simulink model "frt_e"  (R2012b)
(part 3 of 76)

      |     if (t < 0) || (t > 2),
      |         problem = t;
      |         ctr = numios + 1;
      |     end
      | end
      | if problem ~= 0,
      |     error('Type cannot be %i, must be 0, 1 or 2.', problem);
      | end
      mask Callback bin_pts:
      | blk = gcb;
      | mode = get_param(blk, 'mode');
      | current_bins = eval(get_param(blk, 'bin_pts'));
      | if (strcmp(mode, 'one value') || strcmp(mode, 'fields of equal size')) && (length(current_bins) > 1),
      |     error('Only one binary pt may be specified for this mode.');
      | elseif strcmp(mode, 'fields of arbitrary size')
      |     current_names = textscan(strtrim(strrep(strrep(get_param(blk, 'names'), ']', ''), '[', '')), '%s');
      |     current_names = current_names{1};
      |     numios = length(current_names);
      |     if length(current_bins) ~= numios,
      |         error('%d field names specified, but %d binary pts?', numios, length(current_bins));
      |     end
      | end
  txip3 : Subsystem  Tag=xps:sw_reg  AncestorBlock=xps_library/software register  mask(swreg){mode=one value, io_dir=To Processor, io_delay=0, sample_period=1, names=ip, bitwidths=32, arith_types=0, bin_pts=0, sim_port=off, show_format=on}
      mask prompts: io_dir "I/O direction"; io_delay "I/O delay"; sample_period "Sample period"; names "Name:"; bitwidths "Bitwidth:"; arith_types "Type (ufix=0, fix=1, bool=2):"; bin_pts "Binary pt:"; sim_port "Provide sim input/output?"; show_format "Print format string?"
      mask init:
      | swreg_init(gcb)
      settings: AttributesFormatString=1output:uf32.0,
      mask TypeOptions mode: one value | fields of equal size | fields of arbitrary size
      mask Callback mode: swreg_cb(gcb);
      mask TypeOptions io_dir: To Processor | From Processor
      mask Callback io_dir:
      | mask_enables = get_param(gcb, 'MaskEnables');
      | mask_names = get_param(gcb, 'MaskNames');
      | if strcmp(get_param(gcb, 'io_dir'), 'To Processor'),
      |     mask_enables{ismember(mask_names, 'sample_period')} = 'off';
      | else
      |     mask_enables{ismember(mask_names, 'sample_period')} = 'on';
      | end
      | set_param(gcb, 'MaskEnables', mask_enables);
      mask Callback bitwidths:
      | blk = gcb;
      | mode = get_param(blk, 'mode');
      | current_widths = eval(get_param(blk, 'bitwidths'));
      | if (strcmp(mode, 'one value') || strcmp(mode, 'fields of equal size')) && (length(current_widths) > 1),
      |     error('Only one width may be specified for this mode.');
      | elseif strcmp(mode, 'fields of arbitrary size')
      |     current_names = textscan(strtrim(strrep(strrep(get_param(blk, 'names'), ']', ''), '[', '')), '%s');
      |     current_names = current_names{1};
      |     numios = length(current_names);
      |     if length(current_widths) ~= numios,
      |         error('%d field names specified, but %d widths?', numios, length(current_widths));
      |     end
      | end
      | total_width = 0;
      | for ctr = 1 : length(current_widths),
      |     total_width = total_width + current_widths(ctr);
      | end
      | if total_width > 32,
      |     error('Total width must be 32 or less, set to %d.', total_width);
      | end
      mask Callback arith_types:
      | blk = gcb;
      | mode = get_param(blk, 'mode');
      | current_types = eval(get_param(blk, 'arith_types'));
      | numios = length(current_types);
      | if (strcmp(mode, 'one value') || strcmp(mode, 'fields of equal size')) && (length(current_types) > 1),
      |     error('Only one type may be specified for this mode.');
      | elseif strcmp(mode, 'fields of arbitrary size')
      |     current_names = textscan(strtrim(strrep(strrep(get_param(blk, 'names'), ']', ''), '[', '')), '%s');
      |     current_names = current_names{1};
      |     numios = length(current_names);
      |     if length(current_types) ~= numios,
      |         error('%d field names specified, but %d types?', numios, length(current_types));
      |     end
      | end
      | problem = 0;
      | for ctr = 1 : numios,
      |     t = current_types(ctr);
      |     if (t < 0) || (t > 2),
      |         problem = t;
      |         ctr = numios + 1;
      |     end
      | end
      | if problem ~= 0,
      |     error('Type cannot be %i, must be 0, 1 or 2.', problem);
      | end
      mask Callback bin_pts:
      | blk = gcb;
      | mode = get_param(blk, 'mode');
      | current_bins = eval(get_param(blk, 'bin_pts'));
      | if (strcmp(mode, 'one value') || strcmp(mode, 'fields of equal size')) && (length(current_bins) > 1),
      |     error('Only one binary pt may be specified for this mode.');
      | elseif strcmp(mode, 'fields of arbitrary size')
      |     current_names = textscan(strtrim(strrep(strrep(get_param(blk, 'names'), ']', ''), '[', '')), '%s');
      |     current_names = current_names{1};
      |     numios = length(current_names);
      |     if length(current_bins) ~= numios,
      |         error('%d field names specified, but %d binary pts?', numios, length(current_bins));
      |     end
      | end
  txpport01 : Subsystem  Tag=xps:sw_reg  AncestorBlock=xps_library/software register  mask(swreg){mode=fields of equal size, io_dir=To Processor, io_delay=0, sample_period=1, names=[port0 port1], bitwidths=32/2, arith_types=0, bin_pts=0, sim_port=off, show_format=on}
      mask prompts: io_dir "I/O direction"; io_delay "I/O delay"; sample_period "Sample period"; names "Names [msb ... lsb]:"; bitwidths "Bitwidth:"; arith_types "Type (ufix=0, fix=1, bool=2):"; bin_pts "Binary pt:"; sim_port "Provide sim input/output?"; show_format "Print format string?"
      mask init:
      | swreg_init(gcb)
      settings: AttributesFormatString=2 outputs:uf16.0,uf16.0,
      mask TypeOptions mode: one value | fields of equal size | fields of arbitrary size
      mask Callback mode: swreg_cb(gcb);
      mask TypeOptions io_dir: To Processor | From Processor
      mask Callback io_dir:
      | mask_enables = get_param(gcb, 'MaskEnables');
      | mask_names = get_param(gcb, 'MaskNames');
      | if strcmp(get_param(gcb, 'io_dir'), 'To Processor'),
      |     mask_enables{ismember(mask_names, 'sample_period')} = 'off';
      | else
      |     mask_enables{ismember(mask_names, 'sample_period')} = 'on';
      | end
      | set_param(gcb, 'MaskEnables', mask_enables);
      mask Callback bitwidths:
      | blk = gcb;
      | mode = get_param(blk, 'mode');
      | current_widths = eval(get_param(blk, 'bitwidths'));
      | if (strcmp(mode, 'one value') || strcmp(mode, 'fields of equal size')) && (length(current_widths) > 1),
      |     error('Only one width may be specified for this mode.');
      | elseif strcmp(mode, 'fields of arbitrary size')
      |     current_names = textscan(strtrim(strrep(strrep(get_param(blk, 'names'), ']', ''), '[', '')), '%s');
      |     current_names = current_names{1};
      |     numios = length(current_names);
      |     if length(current_widths) ~= numios,
      |         error('%d field names specified, but %d widths?', numios, length(current_widths));
      |     end
      | end
      | total_width = 0;
      | for ctr = 1 : length(current_widths),
      |     total_width = total_width + current_widths(ctr);
      | end
      | if total_width > 32,
      |     error('Total width must be 32 or less, set to %d.', total_width);
      | end
      mask Callback arith_types:
      | blk = gcb;
      | mode = get_param(blk, 'mode');
      | current_types = eval(get_param(blk, 'arith_types'));
      | numios = length(current_types);
      | if (strcmp(mode, 'one value') || strcmp(mode, 'fields of equal size')) && (length(current_types) > 1),
      |     error('Only one type may be specified for this mode.');
      | elseif strcmp(mode, 'fields of arbitrary size')
      |     current_names = textscan(strtrim(strrep(strrep(get_param(blk, 'names'), ']', ''), '[', '')), '%s');
      |     current_names = current_names{1};
      |     numios = length(current_names);
      |     if length(current_types) ~= numios,
      |         error('%d field names specified, but %d types?', numios, length(current_types));
      |     end
      | end
      | problem = 0;
      | for ctr = 1 : numios,
      |     t = current_types(ctr);
      |     if (t < 0) || (t > 2),
      |         problem = t;
      |         ctr = numios + 1;
      |     end
      | end
      | if problem ~= 0,
      |     error('Type cannot be %i, must be 0, 1 or 2.', problem);
      | end
      mask Callback bin_pts:
      | blk = gcb;
      | mode = get_param(blk, 'mode');
      | current_bins = eval(get_param(blk, 'bin_pts'));
      | if (strcmp(mode, 'one value') || strcmp(mode, 'fields of equal size')) && (length(current_bins) > 1),
      |     error('Only one binary pt may be specified for this mode.');
      | elseif strcmp(mode, 'fields of arbitrary size')
      |     current_names = textscan(strtrim(strrep(strrep(get_param(blk, 'names'), ']', ''), '[', '')), '%s');
      |     current_names = current_names{1};
      |     numios = length(current_names);
      |     if length(current_bins) ~= numios,
      |         error('%d field names specified, but %d binary pts?', numios, length(current_bins));
      |     end
      | end
  txpport23 : Subsystem  Tag=xps:sw_reg  AncestorBlock=xps_library/software register  mask(swreg){mode=fields of equal size, io_dir=To Processor, io_delay=0, sample_period=1, names=[port2 port3], bitwidths=32/2, arith_types=0, bin_pts=0, sim_port=off, show_format=on}
      mask prompts: io_dir "I/O direction"; io_delay "I/O delay"; sample_period "Sample period"; names "Names [msb ... lsb]:"; bitwidths "Bitwidth:"; arith_types "Type (ufix=0, fix=1, bool=2):"; bin_pts "Binary pt:"; sim_port "Provide sim input/output?"; show_format "Print format string?"
      mask init:
      | swreg_init(gcb)
      settings: AttributesFormatString=2 outputs:uf16.0,uf16.0,
      mask TypeOptions mode: one value | fields of equal size | fields of arbitrary size
      mask Callback mode: swreg_cb(gcb);
      mask TypeOptions io_dir: To Processor | From Processor
      mask Callback io_dir:
      | mask_enables = get_param(gcb, 'MaskEnables');
      | mask_names = get_param(gcb, 'MaskNames');
      | if strcmp(get_param(gcb, 'io_dir'), 'To Processor'),
      |     mask_enables{ismember(mask_names, 'sample_period')} = 'off';
      | else
      |     mask_enables{ismember(mask_names, 'sample_period')} = 'on';
      | end
      | set_param(gcb, 'MaskEnables', mask_enables);
      mask Callback bitwidths:
      | blk = gcb;
      | mode = get_param(blk, 'mode');
      | current_widths = eval(get_param(blk, 'bitwidths'));
      | if (strcmp(mode, 'one value') || strcmp(mode, 'fields of equal size')) && (length(current_widths) > 1),
      |     error('Only one width may be specified for this mode.');
      | elseif strcmp(mode, 'fields of arbitrary size')
      |     current_names = textscan(strtrim(strrep(strrep(get_param(blk, 'names'), ']', ''), '[', '')), '%s');
      |     current_names = current_names{1};
      |     numios = length(current_names);
      |     if length(current_widths) ~= numios,
      |         error('%d field names specified, but %d widths?', numios, length(current_widths));
      |     end
      | end
      | total_width = 0;
      | for ctr = 1 : length(current_widths),
      |     total_width = total_width + current_widths(ctr);
      | end
      | if total_width > 32,
      |     error('Total width must be 32 or less, set to %d.', total_width);
      | end
      mask Callback arith_types:
      | blk = gcb;
      | mode = get_param(blk, 'mode');
      | current_types = eval(get_param(blk, 'arith_types'));
      | numios = length(current_types);
      | if (strcmp(mode, 'one value') || strcmp(mode, 'fields of equal size')) && (length(current_types) > 1),
      |     error('Only one type may be specified for this mode.');
      | elseif strcmp(mode, 'fields of arbitrary size')
      |     current_names = textscan(strtrim(strrep(strrep(get_param(blk, 'names'), ']', ''), '[', '')), '%s');
      |     current_names = current_names{1};
      |     numios = length(current_names);
      |     if length(current_types) ~= numios,
      |         error('%d field names specified, but %d types?', numios, length(current_types));
      |     end
      | end
      | problem = 0;
      | for ctr = 1 : numios,
      |     t = current_types(ctr);
      |     if (t < 0) || (t > 2),
      |         problem = t;
      |         ctr = numios + 1;
      |     end
      | end
      | if problem ~= 0,
      |     error('Type cannot be %i, must be 0, 1 or 2.', problem);
      | end
      mask Callback bin_pts:
      | blk = gcb;
      | mode = get_param(blk, 'mode');
      | current_bins = eval(get_param(blk, 'bin_pts'));
      | if (strcmp(mode, 'one value') || strcmp(mode, 'fields of equal size')) && (length(current_bins) > 1),
      |     error('Only one binary pt may be specified for this mode.');
      | elseif strcmp(mode, 'fields of arbitrary size')
      |     current_names = textscan(strtrim(strrep(strrep(get_param(blk, 'names'), ']', ''), '[', '')), '%s');
      |     current_names = current_names{1};
      |     numios = length(current_names);
      |     if length(current_bins) ~= numios,
      |         error('%d field names specified, but %d binary pts?', numios, length(current_bins));
      |     end
      | end
  unpack_and_reorder : Subsystem  mask{n_bits_packet_size=9, n_bits_timestep=9+3, n_bits_fifo_depth=3, n_bits_buffer_depth=3, bram_latency=1}
      mask prompts: n_bits_packet_size "Packet size (2^? 80-bit words after unpacking)"; n_bits_timestep "Packet timestep (2^?)"; n_bits_fifo_depth "FIFO depth (2^? packets)"; n_bits_buffer_depth "Reorder buffer size (2^? packets)"; bram_latency "BRAM latency"
  up_debug : Subsystem  Tag=xps:sw_reg  AncestorBlock=xps_library/software register  mask(swreg){mode=one value, io_dir=From Processor, io_delay=0, sample_period=1, names=gbe_timestep, bitwidths=3, arith_types=0, bin_pts=0, sim_port=off, show_format=on}
      mask prompts: io_dir "I/O direction"; io_delay "I/O delay"; sample_period "Sample period"; names "Name:"; bitwidths "Bitwidth:"; arith_types "Type (ufix=0, fix=1, bool=2):"; bin_pts "Binary pt:"; sim_port "Provide sim input/output?"; show_format "Print format string?"
      mask init:
      | swreg_init(gcb)
      settings: AttributesFormatString=1input:uf3.0,
      mask TypeOptions mode: one value | fields of equal size | fields of arbitrary size
      mask Callback mode: swreg_cb(gcb);
      mask TypeOptions io_dir: To Processor | From Processor
      mask Callback io_dir:
      | mask_enables = get_param(gcb, 'MaskEnables');
      | mask_names = get_param(gcb, 'MaskNames');
      | if strcmp(get_param(gcb, 'io_dir'), 'To Processor'),
      |     mask_enables{ismember(mask_names, 'sample_period')} = 'off';
      | else
      |     mask_enables{ismember(mask_names, 'sample_period')} = 'on';
      | end
      | set_param(gcb, 'MaskEnables', mask_enables);
      mask Callback bitwidths:
      | blk = gcb;
      | mode = get_param(blk, 'mode');
      | current_widths = eval(get_param(blk, 'bitwidths'));
      | if (strcmp(mode, 'one value') || strcmp(mode, 'fields of equal size')) && (length(current_widths) > 1),
      |     error('Only one width may be specified for this mode.');
      | elseif strcmp(mode, 'fields of arbitrary size')
      |     current_names = textscan(strtrim(strrep(strrep(get_param(blk, 'names'), ']', ''), '[', '')), '%s');
      |     current_names = current_names{1};
      |     numios = length(current_names);
      |     if length(current_widths) ~= numios,
      |         error('%d field names specified, but %d widths?', numios, length(current_widths));
      |     end
      | end
      | total_width = 0;
      | for ctr = 1 : length(current_widths),
      |     total_width = total_width + current_widths(ctr);
      | end
      | if total_width > 32,
      |     error('Total width must be 32 or less, set to %d.', total_width);
      | end
      mask Callback arith_types:
      | blk = gcb;
      | mode = get_param(blk, 'mode');
      | current_types = eval(get_param(blk, 'arith_types'));
      | numios = length(current_types);
      | if (strcmp(mode, 'one value') || strcmp(mode, 'fields of equal size')) && (length(current_types) > 1),
      |     error('Only one type may be specified for this mode.');
      | elseif strcmp(mode, 'fields of arbitrary size')
      |     current_names = textscan(strtrim(strrep(strrep(get_param(blk, 'names'), ']', ''), '[', '')), '%s');
      |     current_names = current_names{1};
      |     numios = length(current_names);
      |     if length(current_types) ~= numios,
      |         error('%d field names specified, but %d types?', numios, length(current_types));
      |     end
      | end
      | problem = 0;
      | for ctr = 1 : numios,
      |     t = current_types(ctr);
      |     if (t < 0) || (t > 2),
      |         problem = t;
      |         ctr = numios + 1;
      |     end
      | end
      | if problem ~= 0,
      |     error('Type cannot be %i, must be 0, 1 or 2.', problem);
      | end
      mask Callback bin_pts:
      | blk = gcb;
      | mode = get_param(blk, 'mode');
      | current_bins = eval(get_param(blk, 'bin_pts'));
      | if (strcmp(mode, 'one value') || strcmp(mode, 'fields of equal size')) && (length(current_bins) > 1),
      |     error('Only one binary pt may be specified for this mode.');
      | elseif strcmp(mode, 'fields of arbitrary size')
      |     current_names = textscan(strtrim(strrep(strrep(get_param(blk, 'names'), ']', ''), '[', '')), '%s');
      |     current_names = current_names{1};
      |     numios = length(current_names);
      |     if length(current_bins) ~= numios,
      |         error('%d field names specified, but %d binary pts?', numios, length(current_bins));
      |     end
      | end
  updebug : Subsystem
      mask Display: fprintf('UP\nDEBUG')
  wintime_error : Subsystem  Tag=xps:sw_reg  AncestorBlock=xps_library/software register  mask(swreg){mode=fields of equal size, io_dir=To Processor, io_delay=0, sample_period=1, names=[step vs_spead], bitwidths=16, arith_types=0, bin_pts=0, sim_port=off, show_format=on}
      mask prompts: io_dir "I/O direction"; io_delay "I/O delay"; sample_period "Sample period"; names "Names [msb ... lsb]:"; bitwidths "Bitwidth:"; arith_types "Type (ufix=0, fix=1, bool=2):"; bin_pts "Binary pt:"; sim_port "Provide sim input/output?"; show_format "Print format string?"
      mask init:
      | swreg_init(gcb)
      settings: AttributesFormatString=2 outputs:uf16.0,uf16.0,
      mask TypeOptions mode: one value | fields of equal size | fields of arbitrary size
      mask Callback mode: swreg_cb(gcb);
      mask TypeOptions io_dir: To Processor | From Processor
      mask Callback io_dir:
      | mask_enables = get_param(gcb, 'MaskEnables');
      | mask_names = get_param(gcb, 'MaskNames');
      | if strcmp(get_param(gcb, 'io_dir'), 'To Processor'),
      |     mask_enables{ismember(mask_names, 'sample_period')} = 'off';
      | else
      |     mask_enables{ismember(mask_names, 'sample_period')} = 'on';
      | end
      | set_param(gcb, 'MaskEnables', mask_enables);
      mask Callback bitwidths:
      | blk = gcb;
      | mode = get_param(blk, 'mode');
      | current_widths = eval(get_param(blk, 'bitwidths'));
      | if (strcmp(mode, 'one value') || strcmp(mode, 'fields of equal size')) && (length(current_widths) > 1),
      |     error('Only one width may be specified for this mode.');
      | elseif strcmp(mode, 'fields of arbitrary size')
      |     current_names = textscan(strtrim(strrep(strrep(get_param(blk, 'names'), ']', ''), '[', '')), '%s');
      |     current_names = current_names{1};
      |     numios = length(current_names);
      |     if length(current_widths) ~= numios,
      |         error('%d field names specified, but %d widths?', numios, length(current_widths));
      |     end
      | end
      | total_width = 0;
      | for ctr = 1 : length(current_widths),
      |     total_width = total_width + current_widths(ctr);
      | end
      | if total_width > 32,
      |     error('Total width must be 32 or less, set to %d.', total_width);
      | end
      mask Callback arith_types:
      | blk = gcb;
      | mode = get_param(blk, 'mode');
      | current_types = eval(get_param(blk, 'arith_types'));
      | numios = length(current_types);
      | if (strcmp(mode, 'one value') || strcmp(mode, 'fields of equal size')) && (length(current_types) > 1),
      |     error('Only one type may be specified for this mode.');
      | elseif strcmp(mode, 'fields of arbitrary size')
      |     current_names = textscan(strtrim(strrep(strrep(get_param(blk, 'names'), ']', ''), '[', '')), '%s');
      |     current_names = current_names{1};
      |     numios = length(current_names);
      |     if length(current_types) ~= numios,
      |         error('%d field names specified, but %d types?', numios, length(current_types));
      |     end
      | end
      | problem = 0;
      | for ctr = 1 : numios,
      |     t = current_types(ctr);
      |     if (t < 0) || (t > 2),
      |         problem = t;
      |         ctr = numios + 1;
      |     end
      | end
      | if problem ~= 0,
      |     error('Type cannot be %i, must be 0, 1 or 2.', problem);
      | end
      mask Callback bin_pts:
      | blk = gcb;
      | mode = get_param(blk, 'mode');
      | current_bins = eval(get_param(blk, 'bin_pts'));
      | if (strcmp(mode, 'one value') || strcmp(mode, 'fields of equal size')) && (length(current_bins) > 1),
      |     error('Only one binary pt may be specified for this mode.');
      | elseif strcmp(mode, 'fields of arbitrary size')
      |     current_names = textscan(strtrim(strrep(strrep(get_param(blk, 'names'), ']', ''), '[', '')), '%s');
      |     current_names = current_names{1};
      |     numios = length(current_names);
      |     if length(current_bins) ~= numios,
      |         error('%d field names specified, but %d binary pts?', numios, length(current_bins));
      |     end
      | end
  wintime_snap : Subsystem  Tag=casper:bitsnap  AncestorBlock=casper_library_scopes/bitfield snapshot  mask(bitsnap){io_names=[time36 fengid freqid0], io_widths=[36 4 12], io_bps=[0 0 0], io_types=[0 0 0], snap_storage=bram, snap_dram_dimm=2, snap_dram_clock=250, snap_nsamples=12, snap_data_width=64, snap_offset=on, snap_circap=off, snap_value=off, snap_use_dsp48=on, snap_delay=1, extra_names=[c d], extra_widths=[30 2], extra_bps=[0 0], extra_types=[0 0]}
      mask prompts: io_names "Names [msb...lsb]"; io_widths "Widths [msb...lsb]"; io_bps "Binary pts [msb...lsb]"; io_types "Data types [msb...lsb], ufix=0, fix=1, bool=2"; snap_storage "Storage medium"; snap_dram_dimm "DRAM dimm"; snap_dram_clock "DRAM clock rate"; snap_nsamples "Number of Samples (2^?)"; snap_data_width "Data width"; snap_offset "Start delay support"; snap_circap "Circular capture support"; snap_value "Extra value capture support"; snap_use_dsp48 "Use DSP48s to implement counters"; snap_delay "Pre-snapshot delay"; extra_names "Names [msb...lsb]"; extra_widths "Widths [msb...lsb]"; extra_bps "Binary pts [msb...lsb]"; extra_types "Data types [msb...lsb], ufix=0, fix=1, bool=2"
      mask help:
      | A wrapped snapshot block. Allows specification of inputs to a snapblock word so the toolflow can automatically set up the scope.
      | See documentation for snapshot for explanation of parameters.
      mask init:
      | bitsnap_init(gcb);
      mask TypeOptions snap_storage: bram | dram
      mask Callback snap_storage: bitsnap_callback();
      mask TypeOptions snap_dram_dimm: 1 | 2 | 3 | 4
      mask TypeOptions snap_dram_clock: 200 | 250 | 266 | 300 | 333
      mask TypeOptions snap_data_width: 8 | 16 | 32 | 64 | 128
      mask Callback snap_value: bitsnap_callback();
  xps : xps_library/XSG core config  Tag=xps:xsg  hw_sys=ROACH2:sx475t  clk_src=sys_clk  ROACH_clk_src=adc0_clk  ROACH2_clk_src=sys_clk  MKDIG_clk_src=sys_clk  clk_rate=228  sample_period=1  synthesis_tool=XST
  tag scope: cnt_rst=global, gbe_timestep=global, up_cnt_rst=global, wintime_snap_wesel=global
  wires:
  gbe0/1(led_up) -> Inverter/1, [up_gbe0]
  gbe0/2(led_rx) -> [rx_gbe0]
  gbe0/3(led_tx) -> [tx_gbe0]
  gbe0/5(tx_overflow) -> [tx_over_gbe0], [of_xaui0]
  gbe0/12(rx_overrun) -> [rxover_gbe0]
  gbe0/11(rx_bad_frame) -> [rxbad_gbe0]
  gbe0/6(rx_data) -> [rxdata_gbe0]
  gbe0/7(rx_valid) -> [rxvld_gbe0]
  gbe0/8(rx_source_ip) -> [rxip_gbe0]
  gbe0/9(rx_source_port) -> [rxport_gbe0]
  gbe0/10(rx_end_of_frame) -> [rxeof_gbe0]
  Inverter/1 -> [ldn_xaui0]
  [gbe_rst] -> Delay12/1
  gbe1/1(led_up) -> [up_gbe1], Inverter1/1
  gbe1/2(led_rx) -> [rx_gbe1]
  gbe1/3(led_tx) -> [tx_gbe1]
  gbe1/4(tx_afull) -> [tx_full_gbe1]
  gbe1/5(tx_overflow) -> [tx_over_gbe1], [of_xaui1]
  gbe1/12(rx_overrun) -> [rxover_gbe1]
  gbe1/11(rx_bad_frame) -> [rxbad_gbe1]
  gbe1/6(rx_data) -> [rxdata_gbe1]
  gbe1/7(rx_valid) -> [rxvld_gbe1]
  gbe1/8(rx_source_ip) -> [rxip_gbe1]
  gbe1/9(rx_source_port) -> [rxport_gbe1]
  gbe1/10(rx_end_of_frame) -> [rxeof_gbe1]
  Inverter1/1 -> [ldn_xaui1]
  Delay12/1 -> gbe1/1(rst)
  gbe2/1(led_up) -> [up_gbe2], Inverter3/1
  gbe2/2(led_rx) -> [rx_gbe2]
  gbe2/3(led_tx) -> [tx_gbe2]
  gbe2/4(tx_afull) -> [tx_full_gbe2]
  gbe2/5(tx_overflow) -> [tx_over_gbe2], [of_xaui2]
  gbe2/12(rx_overrun) -> [rxover_gbe2]
  gbe2/11(rx_bad_frame) -> [rxbad_gbe2]
  gbe2/6(rx_data) -> [rxdata_gbe2]
  gbe2/7(rx_valid) -> [rxvld_gbe2]
  gbe2/8(rx_source_ip) -> [rxip_gbe2]
  gbe2/9(rx_source_port) -> [rxport_gbe2]
  gbe2/10(rx_end_of_frame) -> [rxeof_gbe2]
  Inverter3/1 -> [ldn_xaui2]
  gbe3/1(led_up) -> [up_gbe3], Inverter4/1
  gbe3/2(led_rx) -> [rx_gbe3]
  gbe3/3(led_tx) -> [tx_gbe3]
  gbe3/4(tx_afull) -> [tx_full_gbe3]
  gbe3/5(tx_overflow) -> [tx_over_gbe3], [of_xaui3]
  gbe3/12(rx_overrun) -> [rxover_gbe3]
  gbe3/11(rx_bad_frame) -> [rxbad_gbe3]
  gbe3/6(rx_data) -> [rxdata_gbe3]
  gbe3/7(rx_valid) -> [rxvld_gbe3]
  gbe3/8(rx_source_ip) -> [rxip_gbe3]
  gbe3/9(rx_source_port) -> [rxport_gbe3]
  gbe3/10(rx_end_of_frame) -> [rxeof_gbe3]
  Inverter4/1 -> [ldn_xaui3]
  gbe0/4(tx_afull) -> [tx_full_gbe0]
  bus_expand1/2(lsb_out1) -> aligned/2, misaligned/2
  bus_expand1/1(msb_out2) -> misaligned/1, aligned/1
  aligned/1 -> Register4/1
  misaligned/1 -> Register5/1
  [clr_status] -> Register5/2, Register4/2
  Register5/1 -> [data_misaligned]
  Register4/1 -> [data_aligned]
  edge_detect3/1(out) -> pipeline4/1(d)
  edge_detect4/1(out) -> pipeline3/1(d)
  edge_detect5/1(out) -> pipeline2/1(d)
  [unpack_en] -> Register5/3, Register4/3
  [unpack_recvd] -> bus_expand1/1(bus_in)
  Delay8/1 -> [unpack_d80]
  Delay59/1 -> [unpack_en]  "re80_v"
  Delay62/1 -> aligned1/1
  Delay71/1 -> aligned1/2
  Delay78/1 -> [unpack_recvd]
  [sys_rst] -> edge_detect9/1(in)
  [rxdata_gbe0] -> concat0/1
  [rxdata_gbe1] -> concat0/2
  [rxdata_gbe2] -> concat0/3
  [rxdata_gbe3] -> concat0/4
  [rxeof_gbe0] -> concat1/1
  [rxeof_gbe1] -> concat1/2
  [rxeof_gbe2] -> concat1/3
  [rxeof_gbe3] -> concat1/4
  [rxvld_gbe0] -> concat3/1
  [rxvld_gbe1] -> concat3/2
  [rxvld_gbe2] -> concat3/3
  [rxvld_gbe3] -> concat3/4
  bus_expand2/1(msb_out2) -> Delay62/1
  bus_expand2/2(lsb_out1) -> Delay71/1
  control/2(in_arm) -> edge_detect5/1(in)
  Delay82/1 -> [unpack_timestamp]  "tstamp"
  control/13(in_cnt_rst) -> edge_detect1/1(in)
  concat0/1 -> Delay30/1
  concat1/1 -> Delay31/1
  concat3/1 -> Delay32/1
  constant/1 -> unpack_and_reorder/5(transmit)
  unpack_and_reorder/4(timestamp) -> Delay82/1
  unpack_and_reorder/5(recvd) -> Delay78/1
  unpack_and_reorder/6(of_count) -> bus_expand2/1(bus_in)
  unpack_and_reorder/1(sync) -> Delay41/1
  unpack_and_reorder/7(fifo_of) -> [unpack_fifo_or]
  edge_detect1/1(out) -> pipeline14/1(d)
  control/4(in_gbe_rst) -> pipeline5/1(d)
  control/1(in_sys_rst) -> pipeline/1(d)
  Constant4/1 -> gbe1/8(rx_overrun_ack), gbe1/7(rx_ack)
  [gbe_rst] -> Delay10/1
  Delay10/1 -> gbe2/1(rst)
  Constant23/1 -> gbe2/8(rx_overrun_ack), gbe2/7(rx_ack)
  [gbe_rst] -> Delay11/1
  Delay11/1 -> gbe3/1(rst)
  Constant33/1 -> gbe3/8(rx_overrun_ack), gbe3/7(rx_ack)
  [gbe_rst] -> Delay14/1
  [s64_d0] -> Delay24/1
  [s64_ip] -> Delay25/1
  [s64_port] -> Delay26/1
  Logical2/1 -> gbe0/3(tx_valid)
  Constant20/1 -> gbe0/8(rx_overrun_ack), gbe0/7(rx_ack)
  [gbe_cnt_rst] -> Delay47/1
  [gbe_cnt_rst] -> Delay46/1
  [gbe_cnt_rst] -> Delay45/1
  [gbe_cnt_rst] -> Delay44/1
  [gbe_txen] -> Logical4/2, Logical2/2
  [s64_v0] -> Logical2/1
  [s64_d1] -> Delay27/1
  [s64_ip] -> Delay28/1
  [s64_port] -> Delay33/1
  [gbe_txen] -> Logical3/2, Logical7/2
  [s64_v1] -> Logical7/1
  Logical7/1 -> gbe1/3(tx_valid)
  [s64_d2] -> Delay35/1
  [s64_ip] -> Delay36/1
  [s64_port] -> Delay37/1
  [gbe_txen] -> Logical11/2, Logical8/2
  [s64_v2] -> Logical8/1
  [s64_d3] -> Delay38/1
  [s64_ip] -> Delay39/1
  [s64_port] -> Delay40/1
  [gbe_txen] -> Logical12/2, Logical9/2
  [s64_v3] -> Logical9/1
  Logical8/1 -> gbe2/3(tx_valid)
  Logical9/1 -> gbe3/3(tx_valid)
  Constant10/1 -> iptx_base/1(sim_1)
  iptx_base/1(in_reg) -> Delay20/1
  Constant3/1 -> tx_metadata/1(sim_1)
  tx_metadata/2(in_board_id) -> Delay22/1
  Constant5/1 -> tx_metadata/2(sim_2)
  pipeline/1(q) -> [sys_rst]
  pipeline2/1(q) -> [arm]
  pipeline3/1(q) -> [clr_status]
  pipeline4/1(q) -> [clr_adc_bad]
  pipeline5/1(q) -> [gbe_rst]
  pipeline6/1(q) -> [gbe_txen]
  pipeline8/1(q) -> [adc_protect_disable]
  pipeline9/1(q) -> [tvg_en]
  pipeline10/1(q) -> [ct_tvg]
  pipeline11/1(q) -> [packetiser_tvg]
  pipeline12/1(q) -> [fd_fs_tvg]
  pipeline13/1(q) -> [tvg_adc_en]
  pipeline14/1(q) -> [cnt_rst]
  control/12(in_tvg_adc) -> pipeline13/1(d)
  tx_metadata/1(in_porttx) -> Delay21/1
  unpack_and_reorder/8(packet_of) -> [fifo_pktof]
  Delay29/1 -> unpack_and_reorder/1(rst)
  Delay30/1 -> unpack_and_reorder/2(din)
  Delay31/1 -> unpack_and_reorder/3(eof)
  Delay32/1 -> unpack_and_reorder/4(en)
  Delay44/1 -> gbe3/9(debug_rst)
  Delay45/1 -> gbe2/9(debug_rst)
  Delay46/1 -> gbe1/9(debug_rst)
  Delay47/1 -> gbe0/9(debug_rst)
  edge_detect2/1(out) -> pipeline7/1(d)
  pipeline7/1(q) -> [gbe_cnt_rst]
  control/14(in_gbe_cnt_rst) -> edge_detect2/1(in)
  Logical3/1 -> gbe1/6(tx_end_of_frame)
  [s64_eof1] -> Logical3/1
  Logical4/1 -> gbe0/6(tx_end_of_frame)
  [s64_eof0] -> Logical4/1
  Logical11/1 -> gbe2/6(tx_end_of_frame)
  [s64_eof2] -> Logical11/1
  Logical12/1 -> gbe3/6(tx_end_of_frame)
  [s64_eof3] -> Logical12/1
  Delay14/1 -> gbe0/1(rst)
  edge_detect7/1(out) -> pipeline15/1(d)
  pipeline15/1(q) -> [up_cnt_rst]
  Delay20/1 -> [tx_ip_base]
  Delay21/1 -> [tx_port]
  Delay22/1 -> [tx_board_id]
  Delay24/1 -> gbe0/2(tx_data)
  Delay25/1 -> gbe0/4(tx_dest_ip)
  Delay26/1 -> gbe0/5(tx_dest_port)
  Delay27/1 -> gbe1/2(tx_data)
  Delay28/1 -> gbe1/4(tx_dest_ip)
  Delay33/1 -> gbe1/5(tx_dest_port)
  Delay35/1 -> gbe2/2(tx_data)
  Delay36/1 -> gbe2/4(tx_dest_ip)
  Delay37/1 -> gbe2/5(tx_dest_port)
  Delay38/1 -> gbe3/2(tx_data)
  Delay39/1 -> gbe3/4(tx_dest_ip)
  Delay40/1 -> gbe3/5(tx_dest_port)
  unpack_and_reorder/2(dout) -> Delay8/1
  unpack_and_reorder/3(dvalid) -> Delay59/1
  unpack_and_reorder/9(spead_error) -> Terminator1/1
  unpack_and_reorder/10(discarding) -> Terminator2/1
  unpack_and_reorder/11(timestep_error) -> [timestep_error]
  Constant25/1 -> trigger_level/1(sim_1)
  [d80_adc1] -> trig1/2(adc_data)
  trig1/3(trig) -> [trans_stop_1]
  trig1/2(data) -> [trans_d80_1]
  trig0/2(data) -> [trans_d80_0]
  trig0/3(trig) -> [trans_stop_0]
  [d80_adc0] -> trig0/2(adc_data)
  trig1/1(synco) -> [trans_valid80]
  [sync80] -> Concat6/1
  [time80] -> Slice14/1
  Concat6/1 -> trig0/1(synci)
  trig0/1(synco) -> bus_expand/1(bus_in)
  bus_expand/1(msb_out2) -> [trans_trig]
  Slice14/1 -> Concat6/2
  bus_expand/2(lsb_out1) -> [trans_time]
  [valid80] -> trig1/1(synci)
  trigger_level/1(in_trigger_level) -> pipeline17/1(d)
  [unpack_en] -> en_gen/2(en)
  [unpack_timestamp] -> en_gen/3(time_in)
  en_gen/1(dout) -> sync_gen/1(din)
  sync_gen/1(sync) -> data_tvg1/2(sync_in), data_tvg0/2(sync_in)
  data_tvg0/3(dvalid) -> [valid80]
  data_tvg0/1(sync_out) -> [sync80]
  bus_expand6/2(lsb_out1) -> data_tvg1/3(din)
  data_tvg0/2(dout) -> [d80_adc0]
  [tvg_d80_en] -> en_gen/5(tvg_en)
  pipeline17/1(q) -> trig1/3(trig_pnt), trig0/3(trig_pnt)
  [unpack_d80] -> en_gen/1(din)
  bus_expand6/1(msb_out2) -> data_tvg0/3(din)
  data_tvg0/4(misco) -> [time80]
  sync_gen/5(misco) -> data_tvg1/5(misci)
  data_tvg1/2(dout) -> [d80_adc1]
  data_tvg1/3(dvalid) -> Terminator9/1
  data_tvg1/1(sync_out) -> Terminator4/1
  Concat/1 -> en_gen/4(misci)
  [unpack_adc_or] -> Concat/1
  [data_misaligned] -> Concat/2
  data_tvg1/4(misco) -> bus_expand19/1(bus_in)
  bus_expand19/1(msb_out2) -> [adc_or_flag]
  bus_expand19/2(lsb_out1) -> [missing_flag]
  [tvg_adc_en] -> data_tvg0/1(tvg_en), data_tvg1/1(tvg_en)
  en_gen/3(time_out) -> sync_gen/3(time_in)
  en_gen/2(dvalid) -> sync_gen/2(en)
  en_gen/4(misco) -> Slice20/1, Slice19/1
  Slice19/1 -> sync_gen/4(misci)
  Slice20/1 -> sync_gen/5(relock)
  sync_gen/4(time_out) -> data_tvg0/5(misci)
  sync_gen/2(dout) -> bus_expand6/1(bus_in)
  sync_gen/3(dvalid) -> data_tvg1/4(en), data_tvg0/4(en)
  [timestep_error] -> Concat/3
  Slice/1 -> pipeline16/1(d)
  pipeline16/1(q) -> local_time_lsw/1(out_timestamp_lsw)
  Slice16/1 -> Convert1/1
  pipeline47/1(q) -> local_time_msw/1(out_timestamp_msw)
  Convert1/1 -> pipeline47/1(d)
  Concat2/1 -> Slice16/1, [time80_48], Slice/1
  [time80] -> Concat2/1
  Constant53/1 -> Concat2/2
  control/15(in_unpack_cnt_rst) -> edge_detect7/1(in)
  pipeline18/1(q) -> [snappfb_arm]
  control/17(in_snappfb_arm) -> pipeline18/1(d)
  control/5(in_gbe_txen) -> pipeline6/1(d)
  control/6(in_adc_bad_clr) -> edge_detect3/1(in)
  control/7(in_adc_protect_disable) -> pipeline8/1(d)
  control/8(in_tvg_en) -> pipeline9/1(d)
  control/9(in_tvg_ct) -> pipeline10/1(d)
  control/10(in_tvg_packetiser) -> pipeline11/1(d)
  control/11(in_tvg_fdfs) -> pipeline12/1(d)
  pipeline19/1(q) -> [tvg_d80_en]
  control/20(in_tvg_d80) -> pipeline19/1(d)
  aligned1/1 -> [unpack_adc_or]
  [delay_d0] -> pipeline26/1(d)
  [delay_sync] -> pipeline29/1(d)
  [delay_dv] -> pipeline25/1(d)
  [delay_d1] -> pipeline27/1(d)
  pipeline31/1(q) -> pipeline28/1(d)
  Constant32/1 -> coarse_delay0/1(sim_1)
  Constant19/1 -> phase_offset_delta0/1(sim_1)
  Constant16/1 -> delay_delta0/1(sim_1)
  phase_offset_delta0/1(in_phase_offset_delta) -> Slice3/1
  coarse_delay0/1(in_coarse_delay) -> Slice38/1
  Concat22/1 -> [ld_val0]
  delay_delta0/1(in_delay_delta) -> Slice5/1
  Slice2/1 -> pipeline42/1(d)
  Slice3/1 -> pipeline43/1(d)
  Slice38/1 -> pipeline39/1(d)
  Slice4/1 -> pipeline40/1(d)
  Slice5/1 -> pipeline41/1(d)
  fractional_delay0/1(in_fractional_delay) -> Slice4/1
  Constant14/1 -> fractional_delay0/1(sim_1)
  Constant18/1 -> phase_offset0/1(sim_1)
  phase_offset0/1(in_phase) -> Slice2/1
  Concat3/1 -> [ld_val1]
  fft_shift/1(in_fft_shift) -> pipeline31/1(d)
  coarse_delay3/2(dout0) -> pipeline36/1(d)
  coarse_delay3/3(dvalid) -> pipeline38/1(d)
  [ld_val1] -> tl_cd1/3(load_value)
  [ld_val0] -> tl_cd0/3(load_value)
  [sync80] -> tl_cd1/4(sync_in), tl_cd0/4(sync_in)
  [d80_adc1] -> tl_cd1/5(din)
  [valid80] -> tl_cd1/6(en), tl_cd0/6(en)
  [time80_48] -> tl_cd1/2(current_time), tl_cd0/2(current_time)
  [clr_status] -> tl_cd1/1(rst), tl_cd0/1(rst)
  [d80_adc0] -> tl_cd0/5(din)
  tl_cd0/6(time) -> Terminator/1
  tl_cd1/6(time) -> Terminator3/1
  tl_cd1/2(enable) -> coarse_delay3/5(load_val0)
  tl_cd1/3(sync_out) -> coarse_delay3/1(sync_in)
  tl_cd1/5(dvalid) -> coarse_delay3/3(en)
  tl_cd1/1(value) -> coarse_delay3/4(delay_val0)
  tl_cd0/3(sync_out) -> coarse_delay2/1(sync_in)
  tl_cd0/4(dout) -> coarse_delay2/2(din0)
  tl_cd0/5(dvalid) -> coarse_delay2/3(en)
  tl_cd0/1(value) -> coarse_delay2/4(delay_val0)
  tl_cd0/2(enable) -> coarse_delay2/5(load_val0)
  coarse_delay2/1(sync_out) -> pipeline37/1(d)
  coarse_delay2/2(dout0) -> pipeline1/1(d)
  tl_cd1/4(dout) -> coarse_delay3/2(din0)
  coarse_delay2/3(dvalid) -> Terminator5/1
  coarse_delay3/1(sync_out) -> Terminator7/1
  Constant15/1 -> coarse_delay1/1(sim_1)
  Constant13/1 -> phase_offset_delta1/1(sim_1)
  Constant17/1 -> delay_delta1/1(sim_1)
  phase_offset_delta1/1(in_phase_offset_delta) -> Slice6/1
  coarse_delay1/1(in_coarse_delay) -> Slice8/1
  delay_delta1/1(in_delay_delta) -> Slice15/1
  Slice1/1 -> pipeline23/1(d)
  Slice6/1 -> pipeline24/1(d)
  Slice8/1 -> pipeline20/1(d)
  Slice13/1 -> pipeline21/1(d)
  Slice15/1 -> pipeline22/1(d)
  fractional_delay1/1(in_fractional_delay) -> Slice13/1
  Constant12/1 -> fractional_delay1/1(sim_1)
  Constant21/1 -> phase_offset1/1(sim_1)
  phase_offset1/1(in_phase) -> Slice1/1
  pipeline39/1(q) -> Concat22/1
  pipeline40/1(q) -> Concat22/2
  pipeline41/1(q) -> Concat22/3
  pipeline42/1(q) -> Concat22/4
  pipeline43/1(q) -> Concat22/5
  pipeline24/1(q) -> Concat3/5
  pipeline22/1(q) -> Concat3/3
  pipeline23/1(q) -> Concat3/4
  pipeline20/1(q) -> Concat3/1
  pipeline21/1(q) -> Concat3/2
  pipeline37/1(q) -> [delay_sync]
  pipeline1/1(q) -> [delay_d0]
  pipeline36/1(q) -> [delay_d1]
  pipeline38/1(q) -> [delay_dv]
  Convert2/1 -> [pfb_dv]
  Convert3/1 -> [pfb_sync]
  [q_sync] -> generate_pkt_sync/1(sync)
  [q_dv] -> generate_pkt_sync/2(valid)
  concat2/1 -> generate_pkt_sync/3(data)
  [q_d64_0] -> concat2/1
  [q_d64_1] -> concat2/2
  generate_pkt_sync/4(packet_sync) -> [tq_pktsync]
  generate_pkt_sync/1(out_sync) -> [tq_sync]
  generate_pkt_sync/2(out_valid) -> [tq_dv]
  pipeline29/1(q) -> pfb/1
  pipeline28/1(q) -> pfb/5
  pipeline25/1(q) -> pfb/2
  pipeline26/1(q) -> pfb/3
  pipeline27/1(q) -> pfb/4
  pfb/1 -> Convert3/1
  pfb/2 -> Convert2/1
  pfb/3 -> [pfb_d144_0]
  pfb/4 -> [pfb_d144_1]
  pfb/5 -> [pfb_of]
  Counter1/1 -> eq1/1(addr)
  Constant9/1 -> eq1/2(data_in)
  Constant11/1 -> eq1/3(we)
  Delay17/1 -> quant1/1(sync_in)
  Delay16/1 -> quant1/2(din)
  eq1/1(data_out) -> quant1/4(coeffs)
  Delay18/1 -> quant1/3(en)
  [pfb_sync] -> Counter1/1, Delay17/1
  [pfb_d144_1] -> Delay16/1
  [pfb_dv] -> Counter1/2, Delay18/1
  Counter2/1 -> eq0/1(addr)
  Constant22/1 -> eq0/2(data_in)
  Constant24/1 -> eq0/3(we)
  Delay2/1 -> quant0/1(sync_in)
  Delay5/1 -> quant0/2(din)
  Delay1/1 -> quant0/3(en)
  eq0/1(data_out) -> quant0/4(coeffs)
  [pfb_dv] -> Counter2/2, Delay1/1
  [pfb_sync] -> Counter2/1, Delay2/1
  [pfb_d144_0] -> Delay5/1
  quant0/1(sync_out) -> [q_sync]
  quant0/2(dout) -> [q_d64_0]
  quant0/3(dvalid) -> [q_dv]
  quant0/4(of) -> [q_of]
  quant1/2(dout) -> [q_d64_1]
  generate_pkt_sync/3(out_data) -> [tq_d]
  ct/1(sync_out) -> [ct_sync], gap_enforcer/1(sync)  "ctsync"
  gap_enforcer/1(sync_out) -> [gap_sync], flag_fifo/4(rd_sync_in)  "gapsync"
  gap_enforcer/2(dvalid) -> flag_fifo/5(rd_valid)  "gapdata"
  [ctin_dv] -> flag_fifo/2(wr_valid)
  [ctin_sync] -> flag_fifo/1(wr_sync)
  flag_fifo/1(sync) -> [flag_sync], Delay3/1
  flag_fifo/2(valid) -> Delay4/1
  flag_fifo/3(data) -> Delay6/1
  Constant39/1 -> pack/6(flag)
  [tx_board_id] -> pack/7(board_id)
  [sys_rst] -> edge_detect10/1(in)
  [tx_ip_base] -> pack/8(base_ip)
  [tx_port] -> pack/9(base_port)
  gap_enforcer/3(dout) -> flag_fifo/6(rd_data_in)  "gapvalid"
  pack/1(dout) -> Delay23/1  "d"
  pack/2(dvalid) -> Delay7/1  "v"
  pack/3(eof) -> Delay13/1  "e"
  pack/4(overflow) -> Delay9/1  "of"
  pack/5(destination_ip) -> Delay63/1  "dest_ip"
  pack/6(destination_port) -> Delay64/1  "port"
  [ctin_time36] -> flag_fifo/3(wr_flags)  "gap_time"
  Delay23/1 -> bus_expand3/1(bus_in), bus_expand5/1(bus_in)
  Delay7/1 -> bus_expand7/1(bus_in)
  Delay13/1 -> bus_expand8/1(bus_in)
  bus_expand5/1(msb_out4) -> [s64_d0]
  bus_expand7/1(msb_out4) -> [s64_v0]
  bus_expand8/1(msb_out4) -> [s64_eof0]
  Delay9/1 -> bus_expand9/1(bus_in)
  bus_expand9/1(msb_out4) -> [s64_of0]
  Delay63/1 -> [s64_ip], Gateway Out1/1
  Delay64/1 -> [s64_port], Gateway Out2/1
  [ctin_sync] -> ct/1(sync)
  [ctin_d64_1] -> ct/4(din1)
  counter14/1 -> Delay65/1
  Delay65/1 -> ct_errcnt/1(out_errcnt0)
  counter15/1 -> Delay66/1
  Delay67/1 -> counter15/1, counter14/1
  slice5/1 -> counter14/2
  slice6/1 -> counter15/2
  counter16/1 -> Delay68/1
  counter17/1 -> Delay69/1
  Delay70/1 -> counter16/1, counter17/1
  slice7/1 -> counter16/2
  slice8/1 -> counter17/2
  Delay72/1 -> ct_cnt/1(out_validcnt)
  counter18/1 -> Delay72/1
  Delay73/1 -> ct_cnt/2(out_synccnt)
  counter19/1 -> Delay73/1
  Gateway Out1/1 -> To Workspace1/1
  Gateway Out2/1 -> To Workspace2/1
  [ctin_dv] -> ct/2(valid)
  [ctin_d64_0] -> ct/3(din0)
  Delay66/1 -> ct_errcnt/2(out_parerrcnt0)
  Delay68/1 -> ct_errcnt/3(out_errcnt1)
  Delay69/1 -> ct_errcnt/4(out_parerrcnt1)
  [s64_ip] -> Delay49/1
  [s64_port] -> Delay50/1
  Delay49/1 -> Register1/1
  Register1/1 -> txip0/1(out_ip)
  Delay50/1 -> Register2/1
  Register2/1 -> txpport01/1(out_port0)
  Delay51/1 -> Register1/2, Register2/2
  [s64_v0] -> Delay51/1
  [s64_ip] -> Delay52/1
  [s64_port] -> Delay53/1
  Delay52/1 -> Register3/1
  Register3/1 -> txip1/1(out_ip)
  Delay53/1 -> Register6/1
  Register6/1 -> txpport01/2(out_port1)
  Delay54/1 -> Register6/2, Register3/2
  [s64_v1] -> Delay54/1
  [s64_ip] -> Delay55/1
  [s64_port] -> Delay56/1
  Delay55/1 -> Register7/1
  Register7/1 -> txip2/1(out_ip)
  Delay56/1 -> Register8/1
  Delay57/1 -> Register7/2, Register8/2
  [s64_v2] -> Delay57/1
  [s64_ip] -> Delay58/1
  [s64_port] -> Delay60/1
  Delay58/1 -> Register9/1
  Register9/1 -> txip3/1(out_ip)
  Delay60/1 -> Register10/1
  Delay61/1 -> Register10/2, Register9/2
  [s64_v3] -> Delay61/1
  Register8/1 -> txpport23/1(out_port2)
  Register10/1 -> txpport23/2(out_port3)
  [cnt_rst] -> Delay34/1
  Delay34/1 -> counter19/1, counter18/1
  [ct_sync] -> counter19/2
  [ct_valid] -> counter18/2
  ct/7(ct_err) -> [ct_err]  "ctdv"
  ct/8(parity_error) -> [ct_parerr]  "cterr"
  [ct_err] -> slice7/1, slice5/1
  [ct_parerr] -> slice8/1, slice6/1
  [cnt_rst] -> Delay70/1, Delay67/1
  ct/2(dvalid) -> gap_enforcer/2(en), [ct_valid]  "ctd0"
  ct/3(dout0) -> Concat1/1  "ctd1"
  ct/4(dout1) -> Concat1/2  "ctd2"
  ct/5(dout2) -> Concat1/3  "ctd3"
  ct/6(dout3) -> Concat1/4  "ct_valid"
  Concat1/1 -> gap_enforcer/3(din)
  Delay15/1 -> pack/1(rst)
  Delay3/1 -> pack/2(sync_in)
  Delay4/1 -> pack/3(en)
  Delay6/1 -> pack/4(din)
  bus_expand5/2(out3) -> [s64_d1]
  bus_expand7/2(out3) -> [s64_v1]
  bus_expand8/2(out3) -> [s64_eof1]
  bus_expand9/2(out3) -> [s64_of1]
  bus_expand5/3(out2) -> [s64_d2]
  bus_expand7/3(out2) -> [s64_v2]
  bus_expand8/3(out2) -> [s64_eof2]
  bus_expand9/3(out2) -> [s64_of2]
  bus_expand5/4(lsb_out1) -> [s64_d3]
  bus_expand7/4(lsb_out1) -> [s64_v3]
  bus_expand8/4(lsb_out1) -> [s64_eof3]
  bus_expand9/4(lsb_out1) -> [s64_of3]
  flag_fifo/4(flags) -> Delay19/1
  flag_fifo/5(error) -> Terminator31/1
  Constant26/1 -> concat8/2
  Delay19/1 -> concat8/1
  concat8/1 -> pack/5(timestamp)
  ct_tvg/4(pol1) -> [cttvg_d1]
  ct_tvg/2(valid_out) -> [cttvg_dv]
  ct_tvg/3(pol0) -> [cttvg_d0]
  ct_tvg/5(time_out) -> [cttvg_time]
  ct_tvg/6(time_error) -> Terminator12/1
  [q_sync] -> concat4/1
  [q_dv] -> concat4/2
  [time80] -> concat4/5
  concat4/1 -> Mux1/2
  ct_tvg/1(sync_out) -> [cttvg_sync]
  [cttvg_sync] -> concat5/1
  [cttvg_dv] -> concat5/2
  [cttvg_d0] -> concat5/3
  [cttvg_d1] -> concat5/4
  [cttvg_time] -> concat5/5
  concat5/1 -> Mux1/3
  Mux1/1 -> bus_expand10/1(bus_in)
  bus_expand10/1(msb_out5) -> [ctin_sync]
  bus_expand10/2(out4) -> [ctin_dv]
  bus_expand10/3(out3) -> [ctin_d64_0]
  bus_expand10/4(out2) -> [ctin_d64_1]
  bus_expand10/5(lsb_out1) -> [ctin_time36]
  [ct_tvg] -> pipeline49/1(d)
  pipeline49/1(q) -> Mux1/1
  quant1/1(sync_out) -> Terminator6/1
  quant1/3(dvalid) -> Terminator8/1
  quant1/4(of) -> Terminator10/1
  control/3(in_status_clr) -> edge_detect4/1(in)
  Delay41/1 -> [unpack_sync]
  Register11/1 -> Slice9/1, Slice7/1
  [time80] -> pipeline54/1(d)
  Slice7/1 -> sync_timestamp_msw/1(out_reg)
  [sync80] -> pipeline52/1(d)
  [valid80] -> pipeline53/1(d)
  Register12/1 -> Logical1/1  "armed"
  Logical1/1 -> Register12/2, Register11/2
  pipeline52/1(q) -> Register12/3, Register12/1
  pipeline53/1(q) -> Logical1/2
  pipeline54/1(q) -> Register11/1
  [valid80] -> pipeline55/1(d)
  pipeline55/1(q) -> Delay42/1, edge_detect13/1(in)
  counter8/1 -> Register13/1
  edge_detect13/1(out) -> counter8/1, Register13/2
  Delay42/1 -> counter8/2
  Slice9/1 -> sync_timestamp_lsw/1(out_time_lsw)
  Register13/1 -> sync_timestamp_lsw/2(out_pkt_size)
  pipeline56/1(q) -> edge_detect14/1(in)
  edge_detect14/1(out) -> counter9/2
  [timestep_error] -> pipeline56/1(d)
  [cnt_rst] -> pipeline57/1(d)
  pipeline57/1(q) -> counter9/1
  pipeline58/1(q) -> edge_detect15/1(in)
  edge_detect15/1(out) -> counter10/2
  [sync80] -> pipeline58/1(d)
  [cnt_rst] -> pipeline51/1(d)
  pipeline51/1(q) -> counter10/1
  pipeline59/1(q) -> edge_detect16/1(in)
  edge_detect16/1(out) -> counter11/2
  [valid80] -> pipeline59/1(d)
  [cnt_rst] -> pipeline60/1(d)
  pipeline60/1(q) -> counter11/1
  counter9/1 -> sync_timestamp_lsw/3(out_tstep_err_ctr)
  counter10/1 -> sync_timestamp_lsw/4(out_sync80_ctr)
  counter11/1 -> sync_timestamp_lsw/5(out_valid80_ctr)
  [time80] -> ct_tvg/3(timestamp)
  [q_dv] -> ct_tvg/2(en)
  [q_sync] -> ct_tvg/1(sync)
  edge_detect12/1(out) -> counter3/2
  pipeline44/1(q) -> counter3/1
  [cnt_rst] -> pipeline44/1(d)
  [ct_sync] -> edge_detect12/1(in)
  edge_detect6/1(out) -> counter4/2
  pipeline45/1(q) -> counter4/1
  [cnt_rst] -> pipeline45/1(d)
  [gap_sync] -> edge_detect6/1(in)
  edge_detect11/1(out) -> counter6/2
  pipeline46/1(q) -> counter6/1
  [cnt_rst] -> pipeline46/1(d)
  [flag_sync] -> edge_detect11/1(in)
  counter7/1 -> pipeline32/1(d)
  edge_detect8/1(out) -> counter7/2
  pipeline30/1(q) -> counter7/1
  [cnt_rst] -> pipeline30/1(d)
  [ctin_sync] -> edge_detect8/1(in)
  counter3/1 -> pipeline33/1(d)
  counter4/1 -> pipeline34/1(d)
  counter6/1 -> pipeline35/1(d)
  pipeline32/1(q) -> sync_ctrs/1(out_cttvg)
  pipeline33/1(q) -> sync_ctrs/2(out_ct)
  pipeline34/1(q) -> sync_ctrs/3(out_gap)
  pipeline35/1(q) -> sync_ctrs/4(out_flags)
  [q_d64_1] -> concat4/4
  [q_d64_0] -> concat4/3
  pack/7(wintime_snap) -> pipeline50/1(d)
  Delay43/1 -> counter5/1, counter2/1
  [cnt_rst] -> Delay43/1
  counter2/1 -> wintime_error/1(out_step)
  pack/8(wintime_error) -> Delay48/1
  Delay48/1 -> counter2/2
  Delay75/1 -> counter5/2
  pack/9(wintime_sp_error) -> Delay75/1
  counter5/1 -> wintime_error/2(out_vs_spead)
  pipeline50/1(q) -> bus_expand4/1(bus_in)
  bus_expand4/1(msb_out5) -> wintime_snap/1(in_time36)
  bus_expand4/2(out4) -> wintime_snap/2(in_fengid)
  bus_expand4/3(out3) -> wintime_snap/3(in_freqid0)
  bus_expand4/4(out2) -> wintime_snap/4(we)
  bus_expand4/5(lsb_out1) -> wintime_snap/5(trig)
  pipeline48/1(q) -> [wintime_snap_wesel]
  control/21(in_wintime_snap_wesel) -> pipeline48/1(d)
  edge_detect9/1(out) -> Delay29/1
  edge_detect10/1(out) -> Delay15/1
  [up_p0_missed_time_ctr] -> Delay76/1(d)
  [up_p1_missed_time_ctr] -> Delay77/1(d)
  [up_p0_missed_time] -> Delay81/1(d)
  [up_p1_missed_time] -> Delay83/1(d)
  Delay81/1(q) -> Slice10/1
  Delay83/1(q) -> Slice11/1
  Delay76/1(q) -> tmiss_ctr/1(out_p0)
  Delay77/1(q) -> tmiss_ctr/2(out_p1)
  [unpack_recvd] -> Slice17/1, Slice12/1
  Inverter2/1 -> Logical5/1
  [unpack_en] -> Logical6/2, Logical5/2
  Logical5/1 -> counter20/2
  [cnt_rst] -> Delay79/1(d)
  counter20/1 -> recverr_ctr/1(out_p0)
  counter21/1 -> mcnt_relock/1(out_reg)
  [mcnt_relock] -> counter21/2
  Slice10/1 -> tmiss_p0/1(out_reg)
  Slice11/1 -> tmiss_p1/1(out_reg)
  counter22/1 -> recverr_ctr/2(out_p1)
  Slice12/1 -> Inverter2/1
  Logical6/1 -> counter22/2
  Slice17/1 -> Inverter5/1
  Inverter5/1 -> Logical6/1
  [up_timestep_error_future] -> counter23/2
  [up_timestep_error_past] -> counter13/2
  Delay79/1(q) -> counter22/1, counter23/1, counter13/1, counter21/1, counter20/1
  counter23/1 -> timestep_ages/1(out_future)
  counter13/1 -> timestep_ages/2(out_past)
  bus_expand12/2(out7) -> snappfb_0/2(in_i0)
  bus_expand12/1(msb_out8) -> snappfb_0/1(in_r0)
  bus_expand12/3(out6) -> snappfb_0/3(in_r1)
  bus_expand12/4(out5) -> snappfb_0/4(in_i1)
  bus_expand12/5(out4) -> snappfb_0/5(in_r2)
  bus_expand12/6(out3) -> snappfb_0/6(in_i2)
  bus_expand12/7(out2) -> snappfb_0/7(in_r3)
  bus_expand12/8(lsb_out1) -> snappfb_1/1(in_i3)
  [tpfb_d] -> pipeline61/1(d)
  pipeline61/1(q) -> bus_expand12/1(bus_in)
  [tpfb_dv] -> pipeline62/1(d)
  pipeline62/1(q) -> snappfb_0/8(we), snappfb_1/2(we)
  [snappfb_arm] -> pipeline63/1(d)
  [tpfb_pktsync] -> pipeline64/1(d)
  pipeline64/1(q) -> oneshot/2(trigger)
  pipeline63/1(q) -> oneshot/1(arm)
  oneshot/1(oneshot) -> snappfb_0/9(trig), snappfb_1/3(trig)
  [pfb_sync] -> pipeline65/1(d)
  [pfb_dv] -> pipeline66/1(d)
  Mux/1 -> generate_pkt_sync1/3(data)
  generate_pkt_sync1/4(packet_sync) -> [tpfb_pktsync]
  generate_pkt_sync1/1(out_sync) -> [tpfb_sync]
  generate_pkt_sync1/2(out_valid) -> [tpfb_dv]
  generate_pkt_sync1/3(out_data) -> [tpfb_d]
  [pfb_d144_0] -> Mux/2
  [pfb_d144_1] -> Mux/3
  [snappfb_dsel] -> Mux/1
  pipeline65/1(q) -> generate_pkt_sync1/1(sync)
  pipeline66/1(q) -> generate_pkt_sync1/2(valid)
  pipeline67/1(q) -> [snappfb_dsel]
  control/18(in_snappfb_dsel) -> pipeline67/1(d)
  bus_expand11/1(msb_out2) -> snapcoarse_0/5(extra_time36_msb)
  bus_expand13/1(msb_out3) -> snapcoarse_0/1(in_p0_80)
  bus_expand13/2(out2) -> snapcoarse_0/2(in_p1_80_msb)
  bus_expand13/3(lsb_out1) -> snapcoarse_1/1(in_p1_80_lsb)
  Constant1/1 -> snapcoarse_1/5(extra_dontcare)
  [snapcoarse_arm] -> Delay85/1
  Delay85/1 -> oneshot1/1(arm)
  Delay74/1 -> oneshot1/2(trigger)
  edge_detect17/1(out) -> Delay74/1
  Concat4/1 -> Delay86/1
  [delay_dv] -> pipeline70/1(d)
  oneshot1/1(oneshot) -> snapcoarse_0/4(trig), snapcoarse_1/3(trig)
  Delay84/1 -> bus_expand11/1(bus_in)
  Delay86/1 -> bus_expand13/1(bus_in)
  Delay87/1 -> snapcoarse_1/2(we), snapcoarse_0/3(we)
  [delay_d1] -> pipeline69/1(d)
  [delay_d0] -> pipeline68/1(d)
  [time80] -> pipeline71/1(d)
  bus_expand11/2(lsb_out1) -> snapcoarse_1/4(extra_time36_lsb)
  pipeline68/1(q) -> Concat4/1
  pipeline69/1(q) -> Concat4/2
  pipeline70/1(q) -> edge_detect17/1(in), Delay87/1
  pipeline71/1(q) -> Delay84/1
  pipeline72/1(q) -> [snapcoarse_arm]
  control/16(in_snapcoarse_arm) -> pipeline72/1(d)
  [tq_d] -> pipeline73/1(d)
  pipeline73/1(q) -> bus_expand14/1(bus_in)
  [tq_dv] -> pipeline74/1(d)
  pipeline74/1(q) -> snapquant/17(we)
  [snapquant_arm] -> pipeline75/1(d)
  [tq_pktsync] -> pipeline76/1(d)
  pipeline76/1(q) -> oneshot2/2(trigger)
  pipeline75/1(q) -> oneshot2/1(arm)
  oneshot2/1(oneshot) -> snapquant/18(trig)
  bus_expand14/5(out12) -> snapquant/5(in_r02)
  bus_expand14/1(msb_out16) -> snapquant/1(in_r00)
  bus_expand14/8(out9) -> snapquant/8(in_i03)
  bus_expand14/10(out7) -> snapquant/10(in_i10)
  bus_expand14/11(out6) -> snapquant/11(in_r11)
  bus_expand14/12(out5) -> snapquant/12(in_i11)
  bus_expand14/13(out4) -> snapquant/13(in_r12)
  bus_expand14/14(out3) -> snapquant/14(in_i12)
  bus_expand14/15(out2) -> snapquant/15(in_r13)
  bus_expand14/16(lsb_out1) -> snapquant/16(in_i13)
  bus_expand14/7(out10) -> snapquant/7(in_r03)
  bus_expand14/3(out14) -> snapquant/3(in_r01)
  bus_expand14/6(out11) -> snapquant/6(in_i02)
  bus_expand14/2(out15) -> snapquant/2(in_i00)
  bus_expand14/9(out8) -> snapquant/9(in_r10)
  bus_expand14/4(out13) -> snapquant/4(in_i01)
  pipeline77/1(q) -> [snapquant_arm]
  control/19(in_snapquant_arm) -> pipeline77/1(d)
  [up_gbe0] -> gbe_status/1(out_gbe0_linkup)
  [up_gbe1] -> gbe_status/2(out_gbe1_linkup)
  [up_gbe2] -> gbe_status/3(out_gbe2_linkup)
  [up_gbe3] -> gbe_status/4(out_gbe3_linkup)
  up_debug/1(in_gbe_timestep) -> Delay88/1(d)
  Delay88/1(q) -> [gbe_timestep]
  unpack_and_reorder/12(mcnt_relock) -> [mcnt_relock]
  counter12/1 -> pipeline79/1(d)
  [cnt_rst] -> pipeline78/1(d)
  counter1/1 -> pipeline80/1(d)
  Logical/1 -> counter12/2
  Logical10/1 -> counter1/2
  pipeline78/1(q) -> counter1/1, counter12/1
  [pfb_of] -> bus_expand15/1(bus_in)
  bus_expand15/1(msb_out2) -> edge_detect19/1(in)
  edge_detect19/1(out) -> Logical/1
  edge_detect18/1(out) -> Logical10/1
  [pfb_dv] -> Logical10/2, Logical/2
  bus_expand15/2(lsb_out1) -> edge_detect18/1(in)
  pipeline79/1(q) -> pfb_of/1(out_of0)
  pipeline80/1(q) -> pfb_of/2(out_of1)
